simulink model "Tyler_Nonlinear_Model"  (R2018b)
settings: Solver=VariableStepAuto  StartTime=0.0  StopTime=10.0  RelTol=1e-3
undefined symbols (not defined in the file or in its folder): A_h, a_right, added_mass, b_right, c_heel, d_yaw, I_xx, I_xz, I_zz, k1, m, rho_w, X_u_dot, Y_v_dot
libraries: sailbot_library x4, Sailbots x2
settings Model: Creator=tlum1  LastModifiedBy=brucecui
settings SFSimCC: SimUseLocalCustomCode=off
settings RTWCC: RTWUseLocalCustomCode=off
settings CodeAppCC: StateflowObjectComments=on

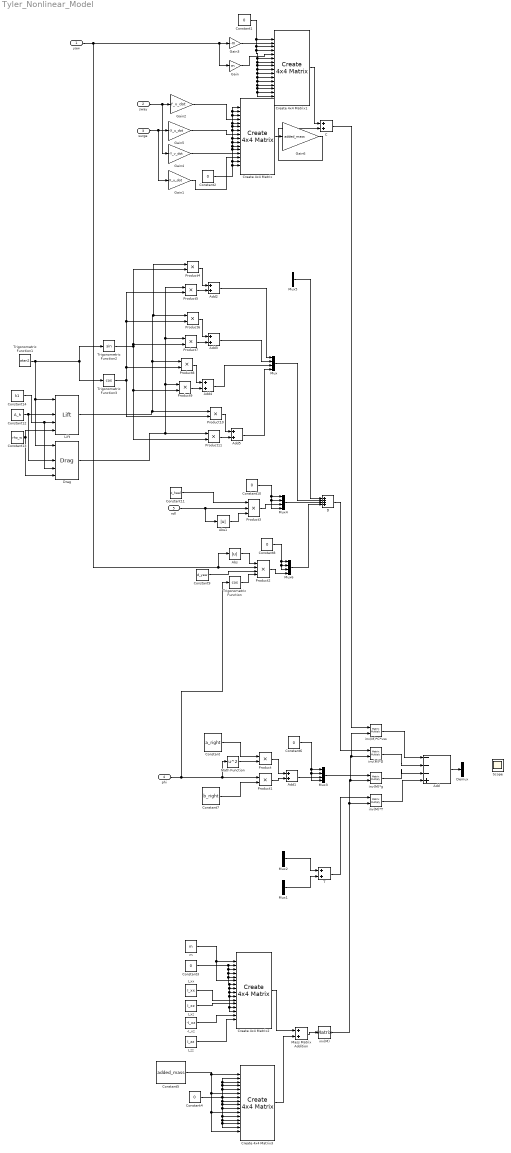
== system Tyler_Nonlinear_Model ==
  yaw : Inport
  sway : Inport  Port=2
  surge : Inport  Port=3
  phi : Inport  Port=4
  roll : Inport  Port=5
  -I_xz : Constant  Value=-I_xz
  Abs : Abs
  Abs1 : Abs
  Add : Sum  Inputs=---|+
  Add{1..5} (5 alike) : Sum
  C : Sum
  Constant : Constant  Value=a_right
  Constant{1..4,6,8,10} (7 alike) : Constant  Value=0
  Constant11 : Constant  Value=c_heel
  Constant12 : Constant  Value=A_h
  Constant13 : Constant  Value=rho_w
  Constant14 : Constant  Value=k1
  Constant5 : Constant  Value=added_mass
  Constant7 : Constant  Value=b_right
  Constant9 : Constant  Value=d_yaw
  Create 4x4 Matrix{,1..3} (4 alike) : sailbot_library/Create 4x4 Matrix  SystemSampleTime=-1
  D : Sum  Inputs=++++
  Demux : Demux
  Drag : Sailbots/Drag
      settings: SourceProductName=Sailbots
  Gain : Gain  Gain=m
  Gain1 : Gain  Gain=X_u_dot
  Gain2 : Gain  Gain=Y_v_dot
  Gain3 : Gain  Gain=-m
  Gain4 : Gain  Gain=-Y_v_dot
  Gain5 : Gain  Gain=-X_u_dot
  Gain6 : Gain  Gain=added_mass
  I_xx : Constant  Value=I_xx
  I_xz : Constant  Value=I_xz
  I_zz : Constant  Value=I_zz
  Lift : Sailbots/Lift
      settings: SourceProductName=Sailbots
  Mass Matrix Addition : Sum
  Math Function : Math  Operator=square  SaturateOnIntegerOverflow=on
  Mux{,1..6} (7 alike) : Mux
  Product{,1,4..11} (10 alike) : Product
  Product2 : Product  Inputs=4
  Product3 : Product  Inputs=3
  Scope : Scope
  T : Sum
  Trigonometric Function : Trigonometry  Operator=cos
  Trigonometric Function1 : Trigonometry  Operator=atan2
  Trigonometric Function2 : Trigonometry
  Trigonometric Function3 : Trigonometry  Operator=cos
  "inv(M) " : Product  Inputs=1  Multiplication=Matrix(*)  SaturateOnIntegerOverflow=on  RndMeth=Zero
  inv(M)*C*vss : Product  Multiplication=Matrix(*)
  inv(M)*D : Product  Multiplication=Matrix(*)
  inv(M)*T : Product  Multiplication=Matrix(*)
  inv(M)*g : Product  Multiplication=Matrix(*)
  m : Constant  Value=m
  wires:
  inv(M)*D/1 -> Add/2
  inv(M)*g/1 -> Add/3
  inv(M)*C*vss/1 -> Add/1
  Add/1 -> Demux/1
  inv(M)*T/1 -> Add/4
  "inv(M) "/1 -> inv(M)*C*vss/2, inv(M)*D/2, inv(M)*g/2, inv(M)*T/2
  Mass Matrix Addition/1 -> "inv(M) "/1
  C/1 -> inv(M)*C*vss/1
  D/1 -> inv(M)*D/1
  T/1 -> inv(M)*T/1
  Mux2/1 -> T/1
  Mux1/1 -> T/2
  Mux3/1 -> inv(M)*g/1
  Mux6/1 -> D/4
  Mux4/1 -> D/3
  Mux/1 -> D/2
  Mux5/1 -> D/1
  Constant2/1 -> Create 4x4 Matrix/16, Create 4x4 Matrix/15, Create 4x4 Matrix/12, Create 4x4 Matrix/11, Create 4x4 Matrix/10, Create 4x4 Matrix/9, Create 4x4 Matrix/7, Create 4x4 Matrix/6, Create 4x4 Matrix/5, Create 4x4 Matrix/3, Create 4x4 Matrix/1, Create 4x4 Matrix/2
  Constant1/1 -> Create 4x4 Matrix1/1, Create 4x4 Matrix1/3, Create 4x4 Matrix1/4, Create 4x4 Matrix1/6, Create 4x4 Matrix1/7, Create 4x4 Matrix1/8, Create 4x4 Matrix1/9, Create 4x4 Matrix1/10, Create 4x4 Matrix1/11, Create 4x4 Matrix1/12, Create 4x4 Matrix1/13, Create 4x4 Matrix1/14, Create 4x4 Matrix1/15, Create 4x4 Matrix1/16
  Gain/1 -> Create 4x4 Matrix1/5
  Gain2/1 -> Create 4x4 Matrix/4
  Gain1/1 -> Create 4x4 Matrix/14
  Gain3/1 -> Create 4x4 Matrix1/2
  Gain4/1 -> Create 4x4 Matrix/13
  Gain5/1 -> Create 4x4 Matrix/8
  Create 4x4 Matrix2/1 -> Mass Matrix Addition/1
  Create 4x4 Matrix3/1 -> Mass Matrix Addition/2
  Constant3/1 -> Create 4x4 Matrix2/2, Create 4x4 Matrix2/3, Create 4x4 Matrix2/4, Create 4x4 Matrix2/5, Create 4x4 Matrix2/7, Create 4x4 Matrix2/8, Create 4x4 Matrix2/9, Create 4x4 Matrix2/10, Create 4x4 Matrix2/13, Create 4x4 Matrix2/14
  m/1 -> Create 4x4 Matrix2/1, Create 4x4 Matrix2/6
  I_xx/1 -> Create 4x4 Matrix2/11
  I_xz/1 -> Create 4x4 Matrix2/12
  -I_xz/1 -> Create 4x4 Matrix2/15
  I_zz/1 -> Create 4x4 Matrix2/16
  Constant4/1 -> Create 4x4 Matrix3/8, Create 4x4 Matrix3/9, Create 4x4 Matrix3/10, Create 4x4 Matrix3/12, Create 4x4 Matrix3/13, Create 4x4 Matrix3/15, Create 4x4 Matrix3/14, Create 4x4 Matrix3/7, Create 4x4 Matrix3/5, Create 4x4 Matrix3/4, Create 4x4 Matrix3/2, Create 4x4 Matrix3/3
  sway/1 -> Gain4/1, Gain2/1
  surge/1 -> Gain1/1, Gain5/1
  Create 4x4 Matrix/1 -> Gain6/1
  Gain6/1 -> C/2
  Constant5/1 -> Create 4x4 Matrix3/6, Create 4x4 Matrix3/16, Create 4x4 Matrix3/11, Create 4x4 Matrix3/1
  Constant6/1 -> Mux3/1, Mux3/2, Mux3/4
  Add1/1 -> Mux3/3
  Product/1 -> Add1/1
  Product1/1 -> Add1/2
  Constant/1 -> Product/1
  Constant7/1 -> Product1/2
  Math Function/1 -> Product/2
  Constant8/1 -> Mux6/1, Mux6/2, Mux6/3
  Product2/1 -> Mux6/4
  Trigonometric Function/1 -> Product2/4
  phi/1 -> Trigonometric Function/1, Math Function/1, Product1/1
  Abs/1 -> Product2/1
  yaw/1 -> Abs/1, Product2/2, Gain/1, Gain3/1
  Constant9/1 -> Product2/3
  Constant10/1 -> Mux4/1, Mux4/2, Mux4/4
  Product3/1 -> Mux4/3
  Abs1/1 -> Product3/3
  roll/1 -> Abs1/1, Product3/2
  Constant11/1 -> Product3/1
  Add2/1 -> Mux/1
  Product4/1 -> Add2/1
  Product5/1 -> Add2/2
  Product6/1 -> Add3/1
  Product7/1 -> Add3/2
  Add3/1 -> Mux/2
  Product8/1 -> Add4/1
  Product9/1 -> Add4/2
  Product10/1 -> Add5/1
  Product11/1 -> Add5/2
  Add4/1 -> Mux/3
  Add5/1 -> Mux/4
  Lift/1 -> Product4/1, Product6/1, Product8/1, Product10/1
  Drag/1 -> Product5/1, Product7/1, Product9/1, Product11/1
  Trigonometric Function1/1 -> Drag/1, Lift/1, Trigonometric Function3/1, Trigonometric Function2/1
  Trigonometric Function2/1 -> Product9/2, Product11/2, Product7/2, Product4/2
  Trigonometric Function3/1 -> Product10/2, Product8/2, Product6/2, Product5/2
  Constant12/1 -> Drag/3, Lift/3
  Constant13/1 -> Lift/5, Drag/5
  Constant14/1 -> Drag/4, Lift/4
  Create 4x4 Matrix1/1 -> C/1
